simulink model "sldemo_varsize_dataLengthAdaptFixSizeImpl"  (Simulink 7.6)
settings: Solver=FixedStepDiscrete  StartTime=0.0  StopTime=2.0  RelTol=1e-3
libraries: simulink x3
settings Model: Creator=The MathWorks Inc.
settings DataIOCC: SaveFormat=StructureWithTime
settings DebuggingCC: SolverPrmCheckMsg=none
settings SFSimCC: SimParseCustomCode=off

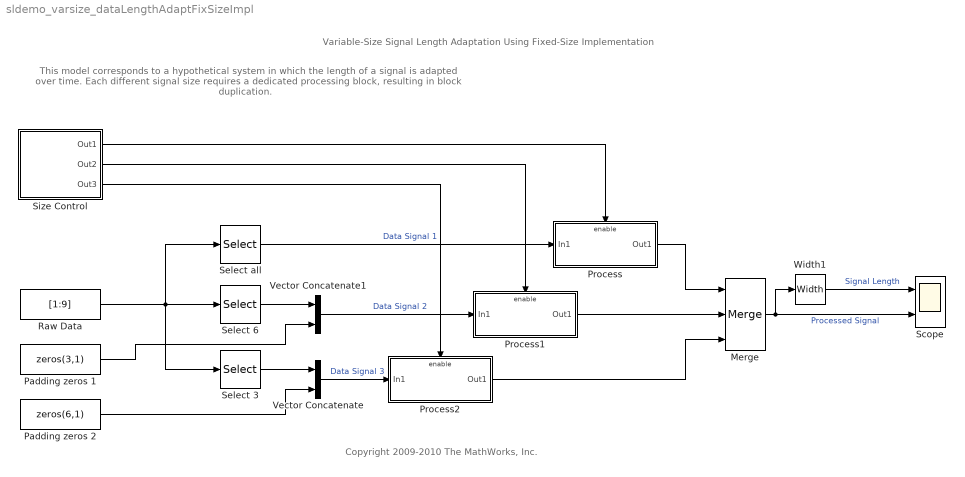
== system sldemo_varsize_dataLengthAdaptFixSizeImpl ==
  note: Copyright 2009-2010 The MathWorks, Inc.
  note: Variable-Size Signal Length Adaptation Using Fixed-Size Implementation
  note: This model corresponds to a hypothetical system in which the length of a signal is adapted over time.
      | Each different signal size requires a dedicated processing block, resulting in block duplication.
  Merge : Merge  Inputs=3  AllowUnequalInputPortWidths=on
  Padding zeros 1 : Constant  Value=zeros(3,1)
  Padding zeros 2 : Constant  Value=zeros(6,1)
  Process : Subsystem  TreatAsAtomicUnit=on
  Process1 : Subsystem  TreatAsAtomicUnit=on
  Process2 : Subsystem  TreatAsAtomicUnit=on
  Raw Data : Constant  Value=[1:9]
  Scope : Scope  NumInputPorts=2
      settings: YMin=17~0  YMax=19~3
  Select 3 : Selector  InputPortWidth=9  IndexOptions=Index vector (dialog)  Indices=1:3  OutputSizes=1
  Select 6 : Selector  InputPortWidth=9  IndexOptions=Index vector (dialog)  Indices=1:6  OutputSizes=1
  Select all : Selector  InputPortWidth=9  IndexOptions=Select all  Indices=[1 3]  OutputSizes=1
  Size Control : Subsystem
  Vector Concatenate : Concatenate  Mode=Vector
  Vector Concatenate1 : Concatenate  Mode=Vector
  Width1 : Width
  wires:
  Raw Data/1 -> Select all/1, Select 6/1, Select 3/1
  Select all/1 -> Process/1(In1)  "Data Signal 1"
  Process/1(Out1) -> Merge/1
  Process1/1(Out1) -> Merge/2
  Process2/1(Out1) -> Merge/3
  Vector Concatenate/1 -> Process2/1(In1)  "Data Signal 3"
  Padding zeros 2/1 -> Vector Concatenate/2
  Select 3/1 -> Vector Concatenate/1
  Select 6/1 -> Vector Concatenate1/1
  Vector Concatenate1/1 -> Process1/1(In1)  "Data Signal 2"
  Padding zeros 1/1 -> Vector Concatenate1/2
  Size Control/2(Out2) -> Process1/Enable
  Size Control/3(Out3) -> Process2/Enable
  Size Control/1(Out1) -> Process/Enable
  Width1/1 -> Scope/1  "Signal Length"
  Merge/1 -> Scope/2, Width1/1  "Processed Signal"

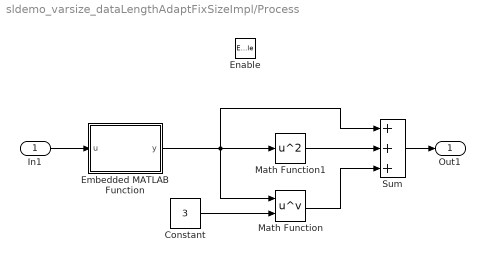
== system sldemo_varsize_dataLengthAdaptFixSizeImpl/Process ==
  In1 : Inport
  Enable : EnablePort  PropagateVarSize=During execution
  Constant : Constant  Value=3
  Embedded MATLAB Function : Stateflow chart  TreatAsAtomicUnit=on
  Math Function : Math  Operator=pow  SaturateOnIntegerOverflow=on
  Math Function1 : Math  Operator=square  SaturateOnIntegerOverflow=on
  Sum : Sum  Inputs=+++
  Out1 : Outport
  wires:
  In1/1 -> Embedded MATLAB Function/1(u)
  Sum/1 -> Out1/1
  Embedded MATLAB Function/1(y) -> Sum/1, Math Function1/1, Math Function/1
  Math Function1/1 -> Sum/2
  Constant/1 -> Math Function/2
  Math Function/1 -> Sum/3

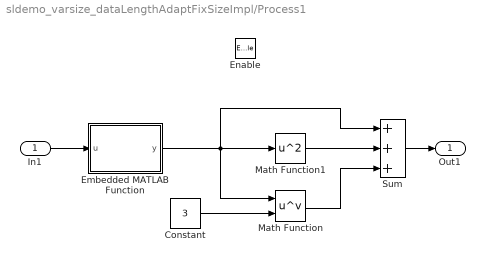
== system sldemo_varsize_dataLengthAdaptFixSizeImpl/Process1 ==
  In1 : Inport
  Enable : EnablePort  PropagateVarSize=During execution
  Constant : Constant  Value=3
  Embedded MATLAB Function : Stateflow chart  TreatAsAtomicUnit=on
  Math Function : Math  Operator=pow  SaturateOnIntegerOverflow=on
  Math Function1 : Math  Operator=square  SaturateOnIntegerOverflow=on
  Sum : Sum  Inputs=+++
  Out1 : Outport
  wires:
  Math Function/1 -> Sum/3
  Constant/1 -> Math Function/2
  Math Function1/1 -> Sum/2
  Embedded MATLAB Function/1(y) -> Math Function/1, Math Function1/1, Sum/1
  Sum/1 -> Out1/1
  In1/1 -> Embedded MATLAB Function/1(u)

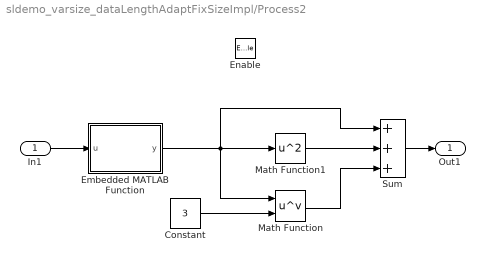
== system sldemo_varsize_dataLengthAdaptFixSizeImpl/Process2 ==
  In1 : Inport
  Enable : EnablePort  PropagateVarSize=During execution
  Constant : Constant  Value=3
  Embedded MATLAB Function : Stateflow chart  TreatAsAtomicUnit=on
  Math Function : Math  Operator=pow  SaturateOnIntegerOverflow=on
  Math Function1 : Math  Operator=square  SaturateOnIntegerOverflow=on
  Sum : Sum  Inputs=+++
  Out1 : Outport
  wires:
  In1/1 -> Embedded MATLAB Function/1(u)
  Sum/1 -> Out1/1
  Embedded MATLAB Function/1(y) -> Sum/1, Math Function1/1, Math Function/1
  Math Function1/1 -> Sum/2
  Constant/1 -> Math Function/2
  Math Function/1 -> Sum/3

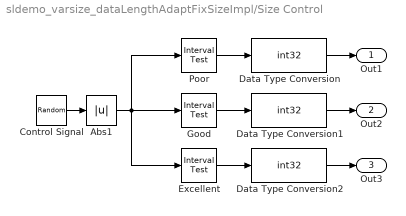
== system sldemo_varsize_dataLengthAdaptFixSizeImpl/Size Control ==
  Abs1 : Abs
  Control Signal : RandomNumber  Variance=0.5  SampleTime=0.1
  Data Type Conversion : DataTypeConversion  OutDataTypeStr=int32
  Data Type Conversion1 : DataTypeConversion  OutDataTypeStr=int32
  Data Type Conversion2 : DataTypeConversion  OutDataTypeStr=int32
  Excellent : simulink/Logic and Bit Operations/Interval Test  SystemSampleTime=-1  IntervalClosedRight=off  uplimit=inf  IntervalClosedLeft=on  lowlimit=0.50  LogicOutDataTypeMode=uint8
  Good : simulink/Logic and Bit Operations/Interval Test  SystemSampleTime=-1  IntervalClosedRight=off  uplimit=0.50  IntervalClosedLeft=on  lowlimit=0.25  LogicOutDataTypeMode=uint8
  Poor : simulink/Logic and Bit Operations/Interval Test  SystemSampleTime=-1  IntervalClosedRight=off  uplimit=0.25  IntervalClosedLeft=on  lowlimit=0.0  LogicOutDataTypeMode=uint8
  Out1 : Outport
  Out2 : Outport  Port=2
  Out3 : Outport  Port=3
  wires:
  Control Signal/1 -> Abs1/1
  Abs1/1 -> Excellent/1, Poor/1, Good/1
  Poor/1 -> Data Type Conversion/1
  Good/1 -> Data Type Conversion1/1
  Excellent/1 -> Data Type Conversion2/1
  Data Type Conversion/1 -> Out1/1
  Data Type Conversion1/1 -> Out2/1
  Data Type Conversion2/1 -> Out3/1

== matlab function Process1/Embedded MATLAB Function ==
  data: u input double size=9; y output double size=18
function y = fcn(u)
%#eml
%
% Insert zeros between elements

sizeU = length(u);
y     = zeros(2*sizeU,1);
for i=1:2*sizeU
    if(mod(i,2))
        y(i)=0; 
    else
        y(i)=u(i/2)/10;
    end
end

== matlab function Process/Embedded MATLAB Function ==
  data: u input double size=9; y output double size=18
function y = fcn(u)
%#eml
%
% Insert zeros between elements

sizeU = length(u);
y     = zeros(2*sizeU,1);
for i=1:2*sizeU
    if(mod(i,2))
        y(i)=0; 
    else
        y(i)=u(i/2)/10;
    end
end

== matlab function Process2/Embedded MATLAB Function ==
  data: u input double size=9; y output double size=18
function y = fcn(u)
%#eml
%
% Insert zeros between elements

sizeU = length(u);
y     = zeros(2*sizeU,1);
for i=1:2*sizeU
    if(mod(i,2))
        y(i)=0; 
    else
        y(i)=u(i/2)/10;
    end
end
